simulink model "Beautiful_powertrain"  (R2024a)
settings: Solver=ode3  StartTime=0.0  StopTime=40  FixedStep=0.001  RelTol=1e-3
model workspace (MAT data in the model file):
  C_Aero_drag = 0.28
  C_rolling_resistance = 0.01
  C_rolling_resitance = 0.01
  C_viscous_damping = 0.02
  Damping_coef = 50
  Gear_ratio = 10
  J_vehicle = 2.56328
  Motor_no_load_speed = 16000
  Motor_rated_load = 150000
  Motor_rated_speed = 9000
  Motor_rotor_damping = 0.02
  Motor_rotor_inertia = 0.05
  Motor_voltage = 450
  Slope = 0
  Vehicle_Wheel_Radius = 0.358
  Vehicle_frontal_area = 2.56
  Vehicle_mass = 2000
values from neighbouring files (symbols this model uses):
  s = sprintf('    [N_diangostic_2.m]
undefined symbols (not defined in the file or in its folder): battery_builder_rtmsupport, gcbh
libraries: Batteries_lib x36, fl_lib x31, nesl_utility x24, ee_lib x3, autolibshared x2, rllib x2, sdl_lib x1
(part 6 of 6)

== system Beautiful_powertrain/Battery/ID4_pack2/ModuleAssembly09 ==
  note: Battery Modules
  note: Output Signals
  ID4_Module : Batteries_lib/Modules/ModuleType1  SOC_vecCell=soc_vec  T_vecCell=T_vec K  V0_matCell=OCV_tbl V  V_rangeCell=V_range V  R0_matCell=R0_tbl Ohm  AHCell=Cap_Ah A*hr  extrapolation_optionCell=simscape.enum.extrapolation.nearest  thermal_massCell=100 J/K  P=3  S=8  iCell_specify=off  iCell_priority=None  iCell=0 A  iCell_nominal_specify=off  iCell_nominal_value=1  iCell_nominal_unit=A  vCell_specify=off  vCell_priority=None  vCell=0 V  vCell_nominal_specify=off  vCell_nominal_value=1  vCell_nominal_unit=V  socCell_specify=on  socCell_priority=High  socCell=SOC_start  socCell_nominal_specify=off  socCell_nominal_value=1  socCell_nominal_unit=1  numCyclesCell_specify=off  numCyclesCell_priority=High  numCyclesCell=0  numCyclesCell_nominal_specify=off  numCyclesCell_nominal_value=1  numCyclesCell_nominal_unit=1  temperatureCell_specify=off  temperatureCell_priority=High  temperatureCell=298.15 K  temperatureCell_nominal_specify=off  temperatureCell_nominal_value=1  temperatureCell_nominal_unit=K  vParallelAssembly_specify=off  vParallelAssembly_priority=None  vParallelAssembly=repmat(0, 8, 1) V  vParallelAssembly_nominal_specify=off  vParallelAssembly_nominal_value=1  vParallelAssembly_nominal_unit=V  socParallelAssembly_specify=off  socParallelAssembly_priority=None  socParallelAssembly=repmat(1, 8, 1)  socParallelAssembly_nominal_specify=off  socParallelAssembly_nominal_value=1  socParallelAssembly_nominal_unit=1
      settings: InternalSimscapePortConfiguration="{\"Bottom\":[{\"id\":\"n\",\"label\":\"-\",\"type\":\"foundation.electrical.electrical\"}],\"Left\":[],\"Right\":[],\"Top\":[{\"id\":\"p\",\"label\":\"+\",\"type\":\"foundation.electrical.electrical\"}]}"
  ID4_Module_outputs : SimscapeProbe  BoundBlock=2521  Variables={iCell, numCyclesCell, socCell, socParallelAssembly, temperatureCell, vCell, vParallelAssembly}
  iCellMux : Mux  Inputs=1
  numCyclesCellMux : Mux  Inputs=1
  socCellMux : Mux  Inputs=1
  socParallelAssemblyMux : Mux  Inputs=1
  temperatureCellMux : Mux  Inputs=1
  vCellMux : Mux  Inputs=1
  vParallelAssemblyMux : Mux  Inputs=1
  + : PMIOPort  Side=Left
  - : PMIOPort  Port=2  Side=Right
  iCell : Outport
  numCyclesCell : Outport  Port=2
  socCell : Outport  Port=3
  socParallelAssembly : Outport  Port=4
  temperatureCell : Outport  Port=5
  vCell : Outport  Port=6
  vParallelAssembly : Outport  Port=7
  wires:
  ID4_Module_outputs/1 -> [iCell1]
  iCellMux/1 -> iCell/1
  [iCell1] -> iCellMux/1
  ID4_Module_outputs/2 -> [numCyclesCell1]
  numCyclesCellMux/1 -> numCyclesCell/1
  [numCyclesCell1] -> numCyclesCellMux/1
  ID4_Module_outputs/3 -> [socCell1]
  socCellMux/1 -> socCell/1
  [socCell1] -> socCellMux/1
  ID4_Module_outputs/4 -> [socParallelAssembly1]
  socParallelAssemblyMux/1 -> socParallelAssembly/1
  [socParallelAssembly1] -> socParallelAssemblyMux/1
  ID4_Module_outputs/5 -> [temperatureCell1]
  temperatureCellMux/1 -> temperatureCell/1
  [temperatureCell1] -> temperatureCellMux/1
  ID4_Module_outputs/6 -> [vCell1]
  vCellMux/1 -> vCell/1
  [vCell1] -> vCellMux/1
  ID4_Module_outputs/7 -> [vParallelAssembly1]
  vParallelAssemblyMux/1 -> vParallelAssembly/1
  [vParallelAssembly1] -> vParallelAssemblyMux/1
  connections:
  ID4_Module/LConn1 -- +/RConn1
  ID4_Module/RConn1 -- -/RConn1

== system Beautiful_powertrain/Battery/ID4_pack2/ModuleAssembly10 ==
  note: Battery Modules
  note: Output Signals
  ID4_Module : Batteries_lib/Modules/ModuleType1  SOC_vecCell=soc_vec  T_vecCell=T_vec K  V0_matCell=OCV_tbl V  V_rangeCell=V_range V  R0_matCell=R0_tbl Ohm  AHCell=Cap_Ah A*hr  extrapolation_optionCell=simscape.enum.extrapolation.nearest  thermal_massCell=100 J/K  P=3  S=8  iCell_specify=off  iCell_priority=None  iCell=0 A  iCell_nominal_specify=off  iCell_nominal_value=1  iCell_nominal_unit=A  vCell_specify=off  vCell_priority=None  vCell=0 V  vCell_nominal_specify=off  vCell_nominal_value=1  vCell_nominal_unit=V  socCell_specify=on  socCell_priority=High  socCell=SOC_start  socCell_nominal_specify=off  socCell_nominal_value=1  socCell_nominal_unit=1  numCyclesCell_specify=off  numCyclesCell_priority=High  numCyclesCell=0  numCyclesCell_nominal_specify=off  numCyclesCell_nominal_value=1  numCyclesCell_nominal_unit=1  temperatureCell_specify=off  temperatureCell_priority=High  temperatureCell=298.15 K  temperatureCell_nominal_specify=off  temperatureCell_nominal_value=1  temperatureCell_nominal_unit=K  vParallelAssembly_specify=off  vParallelAssembly_priority=None  vParallelAssembly=repmat(0, 8, 1) V  vParallelAssembly_nominal_specify=off  vParallelAssembly_nominal_value=1  vParallelAssembly_nominal_unit=V  socParallelAssembly_specify=off  socParallelAssembly_priority=None  socParallelAssembly=repmat(1, 8, 1)  socParallelAssembly_nominal_specify=off  socParallelAssembly_nominal_value=1  socParallelAssembly_nominal_unit=1
      settings: InternalSimscapePortConfiguration="{\"Bottom\":[{\"id\":\"n\",\"label\":\"-\",\"type\":\"foundation.electrical.electrical\"}],\"Left\":[],\"Right\":[],\"Top\":[{\"id\":\"p\",\"label\":\"+\",\"type\":\"foundation.electrical.electrical\"}]}"
  ID4_Module_outputs : SimscapeProbe  BoundBlock=2556  Variables={iCell, numCyclesCell, socCell, socParallelAssembly, temperatureCell, vCell, vParallelAssembly}
  iCellMux : Mux  Inputs=1
  numCyclesCellMux : Mux  Inputs=1
  socCellMux : Mux  Inputs=1
  socParallelAssemblyMux : Mux  Inputs=1
  temperatureCellMux : Mux  Inputs=1
  vCellMux : Mux  Inputs=1
  vParallelAssemblyMux : Mux  Inputs=1
  + : PMIOPort  Side=Left
  - : PMIOPort  Port=2  Side=Right
  iCell : Outport
  numCyclesCell : Outport  Port=2
  socCell : Outport  Port=3
  socParallelAssembly : Outport  Port=4
  temperatureCell : Outport  Port=5
  vCell : Outport  Port=6
  vParallelAssembly : Outport  Port=7
  wires:
  ID4_Module_outputs/1 -> [iCell1]
  iCellMux/1 -> iCell/1
  [iCell1] -> iCellMux/1
  ID4_Module_outputs/2 -> [numCyclesCell1]
  numCyclesCellMux/1 -> numCyclesCell/1
  [numCyclesCell1] -> numCyclesCellMux/1
  ID4_Module_outputs/3 -> [socCell1]
  socCellMux/1 -> socCell/1
  [socCell1] -> socCellMux/1
  ID4_Module_outputs/4 -> [socParallelAssembly1]
  socParallelAssemblyMux/1 -> socParallelAssembly/1
  [socParallelAssembly1] -> socParallelAssemblyMux/1
  ID4_Module_outputs/5 -> [temperatureCell1]
  temperatureCellMux/1 -> temperatureCell/1
  [temperatureCell1] -> temperatureCellMux/1
  ID4_Module_outputs/6 -> [vCell1]
  vCellMux/1 -> vCell/1
  [vCell1] -> vCellMux/1
  ID4_Module_outputs/7 -> [vParallelAssembly1]
  vParallelAssemblyMux/1 -> vParallelAssembly/1
  [vParallelAssembly1] -> vParallelAssemblyMux/1
  connections:
  ID4_Module/LConn1 -- +/RConn1
  ID4_Module/RConn1 -- -/RConn1

== system Beautiful_powertrain/Battery/ID4_pack2/ModuleAssembly11 ==
  note: Battery Modules
  note: Output Signals
  ID4_Module : Batteries_lib/Modules/ModuleType1  SOC_vecCell=soc_vec  T_vecCell=T_vec K  V0_matCell=OCV_tbl V  V_rangeCell=V_range V  R0_matCell=R0_tbl Ohm  AHCell=Cap_Ah A*hr  extrapolation_optionCell=simscape.enum.extrapolation.nearest  thermal_massCell=100 J/K  P=3  S=8  iCell_specify=off  iCell_priority=None  iCell=0 A  iCell_nominal_specify=off  iCell_nominal_value=1  iCell_nominal_unit=A  vCell_specify=off  vCell_priority=None  vCell=0 V  vCell_nominal_specify=off  vCell_nominal_value=1  vCell_nominal_unit=V  socCell_specify=on  socCell_priority=High  socCell=SOC_start  socCell_nominal_specify=off  socCell_nominal_value=1  socCell_nominal_unit=1  numCyclesCell_specify=off  numCyclesCell_priority=High  numCyclesCell=0  numCyclesCell_nominal_specify=off  numCyclesCell_nominal_value=1  numCyclesCell_nominal_unit=1  temperatureCell_specify=off  temperatureCell_priority=High  temperatureCell=298.15 K  temperatureCell_nominal_specify=off  temperatureCell_nominal_value=1  temperatureCell_nominal_unit=K  vParallelAssembly_specify=off  vParallelAssembly_priority=None  vParallelAssembly=repmat(0, 8, 1) V  vParallelAssembly_nominal_specify=off  vParallelAssembly_nominal_value=1  vParallelAssembly_nominal_unit=V  socParallelAssembly_specify=off  socParallelAssembly_priority=None  socParallelAssembly=repmat(1, 8, 1)  socParallelAssembly_nominal_specify=off  socParallelAssembly_nominal_value=1  socParallelAssembly_nominal_unit=1
      settings: InternalSimscapePortConfiguration="{\"Bottom\":[{\"id\":\"n\",\"label\":\"-\",\"type\":\"foundation.electrical.electrical\"}],\"Left\":[],\"Right\":[],\"Top\":[{\"id\":\"p\",\"label\":\"+\",\"type\":\"foundation.electrical.electrical\"}]}"
  ID4_Module_outputs : SimscapeProbe  BoundBlock=2591  Variables={iCell, numCyclesCell, socCell, socParallelAssembly, temperatureCell, vCell, vParallelAssembly}
  iCellMux : Mux  Inputs=1
  numCyclesCellMux : Mux  Inputs=1
  socCellMux : Mux  Inputs=1
  socParallelAssemblyMux : Mux  Inputs=1
  temperatureCellMux : Mux  Inputs=1
  vCellMux : Mux  Inputs=1
  vParallelAssemblyMux : Mux  Inputs=1
  + : PMIOPort  Side=Left
  - : PMIOPort  Port=2  Side=Right
  iCell : Outport
  numCyclesCell : Outport  Port=2
  socCell : Outport  Port=3
  socParallelAssembly : Outport  Port=4
  temperatureCell : Outport  Port=5
  vCell : Outport  Port=6
  vParallelAssembly : Outport  Port=7
  wires:
  ID4_Module_outputs/1 -> [iCell1]
  iCellMux/1 -> iCell/1
  [iCell1] -> iCellMux/1
  ID4_Module_outputs/2 -> [numCyclesCell1]
  numCyclesCellMux/1 -> numCyclesCell/1
  [numCyclesCell1] -> numCyclesCellMux/1
  ID4_Module_outputs/3 -> [socCell1]
  socCellMux/1 -> socCell/1
  [socCell1] -> socCellMux/1
  ID4_Module_outputs/4 -> [socParallelAssembly1]
  socParallelAssemblyMux/1 -> socParallelAssembly/1
  [socParallelAssembly1] -> socParallelAssemblyMux/1
  ID4_Module_outputs/5 -> [temperatureCell1]
  temperatureCellMux/1 -> temperatureCell/1
  [temperatureCell1] -> temperatureCellMux/1
  ID4_Module_outputs/6 -> [vCell1]
  vCellMux/1 -> vCell/1
  [vCell1] -> vCellMux/1
  ID4_Module_outputs/7 -> [vParallelAssembly1]
  vParallelAssemblyMux/1 -> vParallelAssembly/1
  [vParallelAssembly1] -> vParallelAssemblyMux/1
  connections:
  ID4_Module/LConn1 -- +/RConn1
  ID4_Module/RConn1 -- -/RConn1

== system Beautiful_powertrain/Battery/ID4_pack2/ModuleAssembly12 ==
  note: Battery Modules
  note: Output Signals
  ID4_Module : Batteries_lib/Modules/ModuleType1  SOC_vecCell=soc_vec  T_vecCell=T_vec K  V0_matCell=OCV_tbl V  V_rangeCell=V_range V  R0_matCell=R0_tbl Ohm  AHCell=Cap_Ah A*hr  extrapolation_optionCell=simscape.enum.extrapolation.nearest  thermal_massCell=100 J/K  P=3  S=8  iCell_specify=off  iCell_priority=None  iCell=0 A  iCell_nominal_specify=off  iCell_nominal_value=1  iCell_nominal_unit=A  vCell_specify=off  vCell_priority=None  vCell=0 V  vCell_nominal_specify=off  vCell_nominal_value=1  vCell_nominal_unit=V  socCell_specify=on  socCell_priority=High  socCell=SOC_start  socCell_nominal_specify=off  socCell_nominal_value=1  socCell_nominal_unit=1  numCyclesCell_specify=off  numCyclesCell_priority=High  numCyclesCell=0  numCyclesCell_nominal_specify=off  numCyclesCell_nominal_value=1  numCyclesCell_nominal_unit=1  temperatureCell_specify=off  temperatureCell_priority=High  temperatureCell=298.15 K  temperatureCell_nominal_specify=off  temperatureCell_nominal_value=1  temperatureCell_nominal_unit=K  vParallelAssembly_specify=off  vParallelAssembly_priority=None  vParallelAssembly=repmat(0, 8, 1) V  vParallelAssembly_nominal_specify=off  vParallelAssembly_nominal_value=1  vParallelAssembly_nominal_unit=V  socParallelAssembly_specify=off  socParallelAssembly_priority=None  socParallelAssembly=repmat(1, 8, 1)  socParallelAssembly_nominal_specify=off  socParallelAssembly_nominal_value=1  socParallelAssembly_nominal_unit=1
      settings: InternalSimscapePortConfiguration="{\"Bottom\":[{\"id\":\"n\",\"label\":\"-\",\"type\":\"foundation.electrical.electrical\"}],\"Left\":[],\"Right\":[],\"Top\":[{\"id\":\"p\",\"label\":\"+\",\"type\":\"foundation.electrical.electrical\"}]}"
  ID4_Module_outputs : SimscapeProbe  BoundBlock=2626  Variables={iCell, numCyclesCell, socCell, socParallelAssembly, temperatureCell, vCell, vParallelAssembly}
  iCellMux : Mux  Inputs=1
  numCyclesCellMux : Mux  Inputs=1
  socCellMux : Mux  Inputs=1
  socParallelAssemblyMux : Mux  Inputs=1
  temperatureCellMux : Mux  Inputs=1
  vCellMux : Mux  Inputs=1
  vParallelAssemblyMux : Mux  Inputs=1
  + : PMIOPort  Side=Left
  - : PMIOPort  Port=2  Side=Right
  iCell : Outport
  numCyclesCell : Outport  Port=2
  socCell : Outport  Port=3
  socParallelAssembly : Outport  Port=4
  temperatureCell : Outport  Port=5
  vCell : Outport  Port=6
  vParallelAssembly : Outport  Port=7
  wires:
  ID4_Module_outputs/1 -> [iCell1]
  iCellMux/1 -> iCell/1
  [iCell1] -> iCellMux/1
  ID4_Module_outputs/2 -> [numCyclesCell1]
  numCyclesCellMux/1 -> numCyclesCell/1
  [numCyclesCell1] -> numCyclesCellMux/1
  ID4_Module_outputs/3 -> [socCell1]
  socCellMux/1 -> socCell/1
  [socCell1] -> socCellMux/1
  ID4_Module_outputs/4 -> [socParallelAssembly1]
  socParallelAssemblyMux/1 -> socParallelAssembly/1
  [socParallelAssembly1] -> socParallelAssemblyMux/1
  ID4_Module_outputs/5 -> [temperatureCell1]
  temperatureCellMux/1 -> temperatureCell/1
  [temperatureCell1] -> temperatureCellMux/1
  ID4_Module_outputs/6 -> [vCell1]
  vCellMux/1 -> vCell/1
  [vCell1] -> vCellMux/1
  ID4_Module_outputs/7 -> [vParallelAssembly1]
  vParallelAssemblyMux/1 -> vParallelAssembly/1
  [vParallelAssembly1] -> vParallelAssemblyMux/1
  connections:
  ID4_Module/LConn1 -- +/RConn1
  ID4_Module/RConn1 -- -/RConn1

== matlab function Beautiful_powertrain/MATLAB Function2 ==
  data: Vel_ref input; obs output; Vel_act input; u_used input; r output; isdone output
function [obs, r, isdone] = obsReward(Vel_ref, Vel_act, u_used)
%#codegen
% Simple two-element observation and a basic reward.

Vmax = 30;                  % m/s scale (≈108 km/h). Adjust to your use-case.
err  = Vel_ref - Vel_act;

% Normalized observation vector [velocity error; actual velocity]
err_n = max(min(err/Vmax, 1), -1);
v_n   = max(min(Vel_act/Vmax, 1), -1);
obs   = [err_n; v_n];       % 2-by-1 double

% Reward: track speed with small control effort penalty
    % 	1e-3 is a scaling factor: tiny enough not to dominate, but ensures the agent learns to use “just enough” input.
    % 👉 This encourages energy-efficient driving instead of slamming the pedal.

r = -abs(err_n) - 1e-3*(u_used.^2);


% Episode termination condition (optional; keep false for now)
isdone = false;
end

== matlab function Beautiful_powertrain/EV_body/MATLAB Function ==
  data: T_rr output; T_g output; T_d output; T_v output; omega input; T_road output; grade_pct input; Vehicle_mass input; Vehicle_Wheel_Radius input; Cd input; A input; bvis input; Crr input
function [T_rr, T_g, T_d, T_v, T_road] = road_load(omega, grade_pct,Vehicle_mass, Vehicle_Wheel_Radius, Cd, A, bvis, Crr)
%#codegen
% Road-load torque at the WHEEL shaft [N*m]
% Inputs:
%   omega      : wheel angular speed [rad/s]  (from Rotational Motion Sensor)
%   grade_pct  : road grade in percent (e.g., 5 = 5% uphill). Use 0 if unused.
%
% Output:
%   T_road     : resisting torque (opposes motion) [N*m]
vel = omega.*Vehicle_Wheel_Radius;

% ==== Tunable parameters (set to your vehicle) ====
m    = Vehicle_mass;     % vehicle mass [kg]
r    = Vehicle_Wheel_Radius;       % effective wheel radius [m]
g    = 9.81;       % gravity [m/s^2]
rho  = 1.225;      % air density [kg/m^3]
%Cd   = 0.28;       % drag coefficient [-]
%A    = 2.2;        % frontal area [m^2]
%Crr  = 0.012;      % rolling resistance coefficient [-]
%bvis = 1.1;        % viscous/bearing damping [N*m*s/rad]
b_lin =  (bvis / r);
omega0 = 0.5;      % smoothing speed for sign() [rad/s]

% ==== Precompute constants ====
grade = atan(grade_pct/100.0);         % convert % grade to radians
Ka = 0.5 * rho * Cd * A * r;         % aero torque constant [N*m/(rad/s)^2]
Krr = Crr * m * g * r * cos(grade);    % rolling torque magnitude [N*m]
Kg  = m * g * r * sin(grade);          % grade torque magnitude [N*m]

% ==== Smooth sign to avoid chatter near zero speed ====
sgn = tanh(omega/omega0);              % ∈ (-1,1), ~sign(omega)

% ==== Individual torques (opposing motion) ====
T_rr = Krr * sgn;                      % rolling ~ constant with speed
T_g  = Kg  * sgn;                      % grade load
T_d  = Ka  * vel.* abs(vel);      % aero ≈ K * ω^2 * sign(ω)
T_v  = b_lin * vel;                   % viscous (linear with speed)

% ==== Total resisting torque at wheel ====
T_road = -(T_rr + T_g + T_d + T_v);


end

== matlab function Beautiful_powertrain/MATLAB Function1 ==
  data: u input; acc output; brk output
function [acc, brk] = actionMap(u)
% Map agent action u∈[-1,1] -> accelerator duty in [0,1].
% Tune k to make it “more aggressive” without saturating constantly.
u   = max(-1, min(1, u));
k   = 0.6;              % try 0.6 first; 0.8 if it still feels sluggish
acc = min(max(0.5 + k*u, 0), 1);   % -1->0, 0->0.5, +1->1
brk = 0;                % brake disabled for now
end

== matlab function Beautiful_powertrain/MATLAB Function ==
  data: u_scalar input; Acc_cmd output; Brake_cmd output
function [Acc_cmd, Brake_cmd] = actionToPedals(u_scalar)
%#codegen
% Map scalar action u in [-1,1] to plant commands

AccMax  = 1.0;   % set to your plant's full accel command
BrkMax  = 1.0;   % set to your plant's full brake command
Deadband = 0.02; % optional; 0..0.05 is typical

% clamp + deadband
u_scalar = min(max(u_scalar,-1),1);
if abs(u_scalar) < Deadband
    u_scalar = 0;
end

if u_scalar >= 0
    Acc_cmd   = AccMax * u_scalar;     % [0..AccMax]
    Brake_cmd = 0;
else
    Acc_cmd   = 0;
    Brake_cmd = BrkMax * (-u_scalar);  % [0..BrkMax]
end
end
